simulink model "raisedCosineQAM16"  (R2015a)
settings: Solver=ode45  StartTime=0.0  StopTime=10.0  RelTol=1e-3
libraries: commfilt2 x2, commdigbbndam3 x2, commchan3 x1, commsink2 x1, commrandsrc2 x1
settings Model: Creator=maike  LastModifiedBy=maike

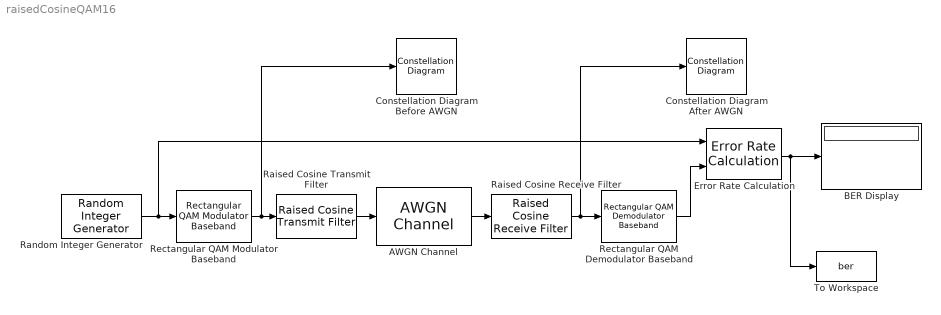
== system raisedCosineQAM16 ==
  AWGN Channel : commchan3/AWGN Channel  InputProcessing=Columns as channels (frame based)  seed=67  noiseMode="Signal to noise ratio  (Eb/No)"  EbNodB=EbNo  EsNodB=10  SNRdB=10  bitsPerSym=4  Ps=1  Tsym=1  variance=1
  BER Display : Display
  Constellation Diagram After AWGN : ConstellationDiagram
  Constellation Diagram Before AWGN : ConstellationDiagram
  Error Rate Calculation : commsink2/Error Rate Calculation  N=10  st_delay=0  cp_mode=Entire frame  subframe=[]  PMode=Port  WsName=ErrorVec  RsMode2=off  stop=off  numErr=100  maxBits=1e6
  Raised Cosine Receive Filter : commfilt2/Raised Cosine Receive Filter  filtType=Square root  N=8  filtSpan=10  currentFiltSpan=10  D=5  R=0.2  sampMode=Mute  saveAsFlag=0  rateMode=Downsampling  downFactor=8  downOffset=0  framing=Enforce single-rate processing  InputProcessing=Columns as channels (frame based)  checkGain=Normalized  filterGain=1  checkCoeff=off  variableName=rcRxFilt  launchFVT=on  roundingMode=Floor  overflowMode=off
  Raised Cosine Transmit Filter : commfilt2/Raised Cosine Transmit Filter  filtType=Square root  filtSpan=10  currentFiltSpan=10  D=5  R=0.2  sampMode=Mute  saveAsFlag=0  N=8  framing=Enforce single-rate processing  InputProcessing=Columns as channels (frame based)  checkGain=Normalized  filterGain=1  checkCoeff=off  variableName=rcTxFilt  launchFVT=on  roundingMode=Floor  overflowMode=off
  Random Integer Generator : commrandsrc2/Random Integer Generator  mul=16  seed=37  Ts=1  frameBased=on  sampPerFrame=100  orient=off  outDataType=double
  Rectangular QAM Demodulator Baseband : commdigbbndam3/Rectangular QAM Demodulator Baseband  M=16  PowType=Min. distance between symbols  MinDist=2  AvgPow=1  PeakPow=1  Ph=0  Dec=Gray  Mapping=[0:15]  OutType=Integer  DecType=Hard decision  VarSource=Dialog  Variance=1  outDtype1=Inherit via internal rule  outDtype2=Inherit via internal rule  derotateFactorWordLen=16  denormFactorWordLen=16  prodOutWordLen=32  prodOutRoundingMode=Floor  prodOutOverflowMode=Wrap  sumWordLen=32
  Rectangular QAM Modulator Baseband : commdigbbndam3/Rectangular QAM Modulator Baseband  M=16  InType=Integer  Enc=Gray  Mapping=[0:15]  PowType=Min. distance between symbols  MinDist=2  AvgPow=1  PeakPow=1  Ph=0  outDtype=double  outWordLen=16  outUDDataType=sfix(16)  outFracLenMode=Best precision  outFracLen=15
  To Workspace : ToWorkspace  VariableName=ber  SampleTime=-1
      settings: MaxDataPoints=2  Save2DSignal=2-D array (concatenate along first dimension)
  wires:
  Random Integer Generator/1 -> Rectangular QAM Modulator Baseband/1, Error Rate Calculation/1
  AWGN Channel/1 -> Raised Cosine Receive Filter/1
  Rectangular QAM Demodulator Baseband/1 -> Error Rate Calculation/2
  Error Rate Calculation/1 -> To Workspace/1, BER Display/1
  Rectangular QAM Modulator Baseband/1 -> Constellation Diagram Before AWGN/1, Raised Cosine Transmit Filter/1
  Raised Cosine Receive Filter/1 -> Rectangular QAM Demodulator Baseband/1, Constellation Diagram After AWGN/1
  Raised Cosine Transmit Filter/1 -> AWGN Channel/1
